simulink model "s8_12"  (Simulink 6.6)
settings: Solver=ode23  SolverMode=SingleTasking  StartTime=0.0  StopTime=t_d  MaxStep=Tc  RelTol=1e-8  AbsTol=1e-8
values from neighbouring files (symbols this model uses):
  F_v = K_r*diag([0.01 0.01])*K_r    [i8_12.m]
  g = 9.81    [i8_12.m]
  K_d = 16*diag([1 1])    [i8_12.m]
  K_p = 100*diag([1 1])    [i8_12.m]
  pi_m = pi_l    [i8_12.m]
  Tc = 0.001    [i8_12.m]
  Ts = Tc    (= 0.001)    [i8_12.m]
undefined symbols (not defined in the file or in its folder): a, iner, iner_l, pi_l, q_i
settings Model: Creator=luigivillani  LastModifiedBy=luigivillani  ExtModeAutoUpdateStatusClock=off
settings SolverCC: InitialStep=0.1*Tc
settings DataIOCC: LimitDataPoints=off  SaveOutput=off  SaveTime=off
settings OptimizationCC: BlockReduction=off  BooleanDataType=off
settings DebuggingCC: SignalResolutionControl=TryResolveAllWithWarning  SolverPrmCheckMsg=none  MultiTaskDSMMsg=warning  MultiTaskCondExecSysMsg=none  StrictBusMsg=None
settings HardwareCC: TargetUnknown=on
settings RTWCC: IncludeERTFirstTime=on

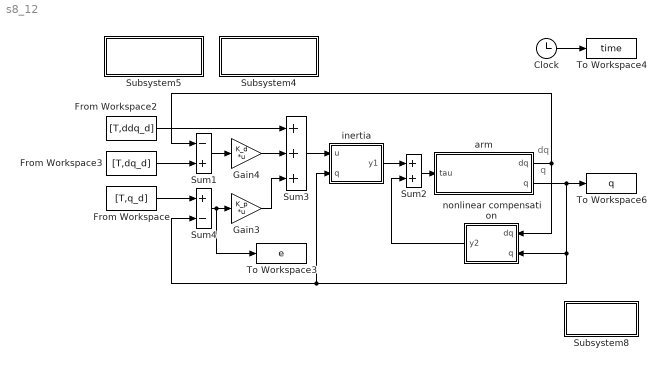
== system s8_12 ==
  note: dq
  note: q
  Clock : Clock
      settings: Decimation=10
  From Workspace : FromWorkspace  VariableName=[T,q_d]  SampleTime=Tc
  From Workspace2 : FromWorkspace  VariableName=[T,ddq_d]  SampleTime=Tc
  From Workspace3 : FromWorkspace  VariableName=[T,dq_d]  SampleTime=Tc
  Gain3 : Gain  Gain=K_p  Multiplication=Matrix(K*u)  SampleTime=Tc
      mask Display: disp('K_p')
  Gain4 : Gain  Gain=K_d  Multiplication=Matrix(K*u)  SampleTime=Tc
      mask Display: disp('K_d')
  Subsystem4 : Subsystem
      settings: OpenFcn=clear all;c=1;i8_12;pi_l=pi_m;
      mask Display: disp('compensated\nload mass')
  Subsystem5 : Subsystem
      settings: OpenFcn=clear all;c=0;i8_12;
      mask Display: disp('noncompensated\nload mass')
  Subsystem8 : Subsystem  Orientation=left
      settings: OpenFcn=p8_12;
      mask Display: disp('plot')
  Sum1 : Sum  Inputs=-+  SampleTime=Tc  SaturateOnIntegerOverflow=on  InputSameDT=on
  Sum2 : Sum  SaturateOnIntegerOverflow=on  InputSameDT=on
  Sum3 : Sum  Inputs=+++  SaturateOnIntegerOverflow=on  InputSameDT=on
  Sum4 : Sum  Inputs=+-  SampleTime=Tc  SaturateOnIntegerOverflow=on  InputSameDT=on
  To Workspace3 : ToWorkspace  VariableName=e  SampleTime=Ts  SaveFormat=Array
      settings: MaxDataPoints=5001
  To Workspace4 : ToWorkspace  VariableName=time  SampleTime=Ts  SaveFormat=Array
      settings: MaxDataPoints=5001
  To Workspace6 : ToWorkspace  VariableName=q  SampleTime=Ts  SaveFormat=Array
      settings: MaxDataPoints=5001
  arm : Subsystem
      mask Display: disp('inv(B(q))(tau-tau'')')
  inertia : Subsystem
      mask Display: disp('B(q)u')
  nonlinear compensation : Subsystem  Orientation=left
      mask Display: disp('n(q,dq)')
  wires:
  Clock/1 -> To Workspace4/1
  Sum2/1 -> arm/1(tau)
  Sum3/1 -> inertia/1(u)
  Gain4/1 -> Sum3/2
  Sum1/1 -> Gain4/1
  From Workspace2/1 -> Sum3/1
  nonlinear compensation/1(y2) -> Sum2/2
  inertia/1(y1) -> Sum2/1
  arm/2("q ") -> To Workspace6/1, Sum4/2, inertia/2(q), nonlinear compensation/2(q)
  From Workspace3/1 -> Sum1/2
  From Workspace/1 -> Sum4/1
  Sum4/1 -> To Workspace3/1, Gain3/1
  arm/1(dq) -> Sum1/1, nonlinear compensation/1(dq)
  Gain3/1 -> Sum3/3

== system s8_12/Subsystem4 ==
  note: start

== system s8_12/Subsystem5 ==
  note: start

== system s8_12/Subsystem8 ==
  note: start

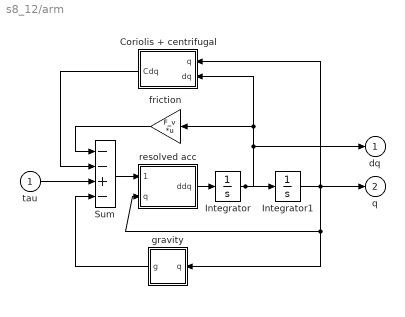
== system s8_12/arm ==
  tau : Inport
  Coriolis + centrifugal : Subsystem  Orientation=left
      mask Display: disp('C(q,dq)dq')
  Integrator : Integrator  InitialCondition=[0 0]  ZeroCross=off
  Integrator1 : Integrator  InitialCondition=q_i  ZeroCross=off
  Sum : Sum  Inputs=--+-  SaturateOnIntegerOverflow=on  InputSameDT=on
  friction : Gain  Orientation=left  Gain=F_v  Multiplication=Matrix(K*u)  SaturateOnIntegerOverflow=on
      mask Display: disp('F_v')
  gravity : Subsystem  Orientation=left
      mask Display: disp('g(q)')
  resolved acc : Subsystem
      mask Display: disp('inv(B(q))')
  dq : Outport  InitialOutput=0
  "q " : Outport  Port=2  InitialOutput=0
  wires:
  Coriolis + centrifugal/1(Cdq) -> Sum/2
  tau/1 -> Sum/3
  Integrator1/1 -> Coriolis + centrifugal/1(q), resolved acc/2(q), gravity/1(q), "q "/1
  resolved acc/1(ddq) -> Integrator/1
  Integrator/1 -> Integrator1/1, dq/1, Coriolis + centrifugal/2(dq), friction/1
  Sum/1 -> resolved acc/1(tau-tau')
  friction/1 -> Sum/1
  gravity/1(g) -> Sum/4

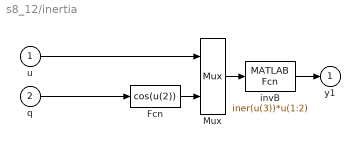
== system s8_12/inertia ==
  u : Inport
  q : Inport  Port=2
  Fcn : Fcn  Expr=cos(u(2))  SampleTime=Tc
  Mux : Mux  Inputs=[2,1]
  "invB " : MATLABFcn  MATLABFcn=iner(u(3))*u(1:2)  OutputDimensions=2  SampleTime=Tc
      mask Display: disp('B(q)')
  y1 : Outport  InitialOutput=0
  wires:
  Fcn/1 -> Mux/2
  "invB "/1 -> y1/1
  Mux/1 -> "invB "/1
  q/1 -> Fcn/1
  u/1 -> Mux/1

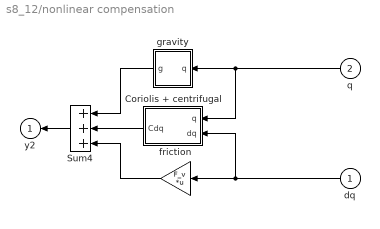
== system s8_12/nonlinear compensation ==
  dq : Inport  Orientation=left
  q : Inport  Orientation=left  Port=2
  Coriolis + centrifugal : Subsystem  Orientation=left
      mask Display: disp('C(q,dq)dq')
  Sum4 : Sum  Orientation=left  Inputs=+++  SaturateOnIntegerOverflow=on  InputSameDT=on
  friction : Gain  Orientation=left  Gain=F_v  Multiplication=Matrix(K*u)  SampleTime=Tc  SaturateOnIntegerOverflow=on
      mask Display: disp('F_v')
  gravity : Subsystem  Orientation=left
      mask Display: disp('g(q)')
  y2 : Outport  Orientation=left  InitialOutput=0
  wires:
  gravity/1(g) -> Sum4/1
  Sum4/1 -> y2/1
  friction/1 -> Sum4/3
  q/1 -> gravity/1(q), Coriolis + centrifugal/1(q)
  dq/1 -> Coriolis + centrifugal/2(dq), friction/1
  Coriolis + centrifugal/1(Cdq) -> Sum4/2

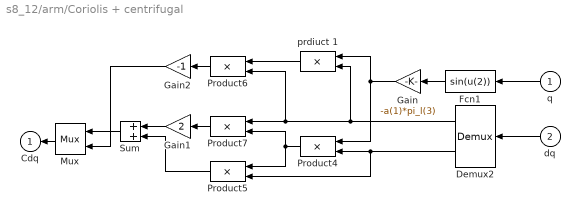
== system s8_12/arm/Coriolis + centrifugal ==
  q : Inport  Orientation=left
  dq : Inport  Orientation=left  Port=2
  Demux2 : Demux  Orientation=left  Outputs=2
  Fcn1 : Fcn  Orientation=left  Expr=sin(u(2))
  Gain : Gain  Orientation=left  Gain=-a(1)*pi_l(3)  SaturateOnIntegerOverflow=on
      mask Display: disp('k_3')
  Gain1 : Gain  Orientation=left  Gain=2  SaturateOnIntegerOverflow=on
  Gain2 : Gain  Orientation=left  Gain=-1  SaturateOnIntegerOverflow=on
  Mux : Mux  Orientation=left  Inputs=2
  Product{4..7} (4 alike) : Product  Orientation=left  SaturateOnIntegerOverflow=on  RndMeth=Zero  InputSameDT=on
  Sum : Sum  Orientation=left  SaturateOnIntegerOverflow=on  InputSameDT=on
  prdiuct 1 : Product  Orientation=left  SaturateOnIntegerOverflow=on  RndMeth=Zero  InputSameDT=on
  Cdq : Outport  Orientation=left  InitialOutput=0
  wires:
  dq/1 -> Demux2/1
  Gain2/1 -> Mux/2
  Product6/1 -> Gain2/1
  Mux/1 -> Cdq/1
  Sum/1 -> Mux/1
  Product5/1 -> Sum/2
  Gain1/1 -> Sum/1
  Product7/1 -> Gain1/1
  Demux2/1 -> prdiuct 1/2, Product6/2, Product7/1
  Demux2/2 -> Product4/2, Product5/2
  prdiuct 1/1 -> Product6/1
  Gain/1 -> prdiuct 1/1, Product4/1
  Fcn1/1 -> Gain/1
  q/1 -> Fcn1/1
  Product4/1 -> Product5/1, Product7/2

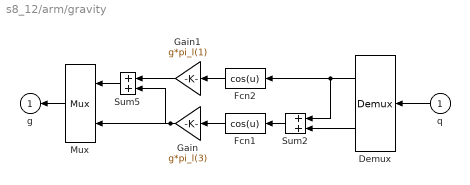
== system s8_12/arm/gravity ==
  q : Inport  Orientation=left
  Demux : Demux  Orientation=left  Outputs=2
  Fcn1 : Fcn  Orientation=left  Expr=cos(u)
  Fcn2 : Fcn  Orientation=left  Expr=cos(u)
  Gain : Gain  Orientation=left  Gain=g*pi_l(3)  SaturateOnIntegerOverflow=on
      mask Display: disp('k_2')
  Gain1 : Gain  Orientation=left  Gain=g*pi_l(1)  SaturateOnIntegerOverflow=on
      mask Display: disp('k_1')
  Mux : Mux  Orientation=left  Inputs=2
  Sum2 : Sum  Orientation=left  SaturateOnIntegerOverflow=on  InputSameDT=on
  Sum5 : Sum  Orientation=left  SaturateOnIntegerOverflow=on  InputSameDT=on
  g : Outport  Orientation=left  InitialOutput=0
  wires:
  q/1 -> Demux/1
  Demux/2 -> Sum2/2
  Sum2/1 -> Fcn1/1
  Fcn1/1 -> Gain/1
  Fcn2/1 -> Gain1/1
  Demux/1 -> Fcn2/1, Sum2/1
  Gain1/1 -> Sum5/1
  Sum5/1 -> Mux/1
  Gain/1 -> Sum5/2, Mux/2
  Mux/1 -> g/1

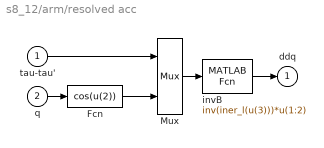
== system s8_12/arm/resolved acc ==
  tau-tau' : Inport
  q : Inport  Port=2
  Fcn : Fcn  Expr=cos(u(2))
  Mux : Mux  Inputs=[2,1]
  "invB " : MATLABFcn  MATLABFcn=inv(iner_l(u(3)))*u(1:2)  OutputDimensions=2
      mask Display: disp('inv(B(q))')
  ddq : Outport  InitialOutput=0
  wires:
  Fcn/1 -> Mux/2
  q/1 -> Fcn/1
  "invB "/1 -> ddq/1
  tau-tau'/1 -> Mux/1
  Mux/1 -> "invB "/1

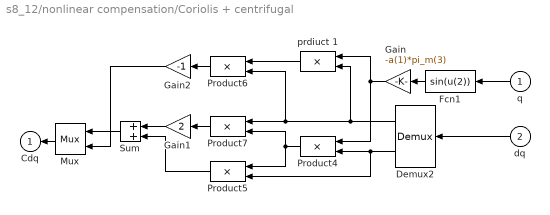
== system s8_12/nonlinear compensation/Coriolis + centrifugal ==
  q : Inport  Orientation=left
  dq : Inport  Orientation=left  Port=2
  Demux2 : Demux  Orientation=left  Outputs=2
  Fcn1 : Fcn  Orientation=left  Expr=sin(u(2))  SampleTime=Tc
  Gain : Gain  Orientation=left  Gain=-a(1)*pi_m(3)  SaturateOnIntegerOverflow=on
      mask Display: disp('k_3')
  Gain1 : Gain  Orientation=left  Gain=2  SaturateOnIntegerOverflow=on
  Gain2 : Gain  Orientation=left  Gain=-1  SaturateOnIntegerOverflow=on
  Mux : Mux  Orientation=left  Inputs=2
  Product{4..7} (4 alike) : Product  Orientation=left  SampleTime=Tc  SaturateOnIntegerOverflow=on  RndMeth=Zero  InputSameDT=on
  Sum : Sum  Orientation=left  SaturateOnIntegerOverflow=on  InputSameDT=on
  prdiuct 1 : Product  Orientation=left  SampleTime=Tc  SaturateOnIntegerOverflow=on  RndMeth=Zero  InputSameDT=on
  Cdq : Outport  Orientation=left  InitialOutput=0
  wires:
  Product4/1 -> Product5/1, Product7/2
  Demux2/1 -> prdiuct 1/2, Product6/2, Product7/1
  Fcn1/1 -> Gain/1
  Gain/1 -> prdiuct 1/1, Product4/1
  prdiuct 1/1 -> Product6/1
  Product7/1 -> Gain1/1
  Gain1/1 -> Sum/1
  Product5/1 -> Sum/2
  Sum/1 -> Mux/1
  Mux/1 -> Cdq/1
  Product6/1 -> Gain2/1
  Gain2/1 -> Mux/2
  q/1 -> Fcn1/1
  dq/1 -> Demux2/1
  Demux2/2 -> Product4/2, Product5/2

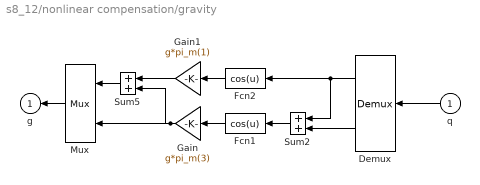
== system s8_12/nonlinear compensation/gravity ==
  q : Inport  Orientation=left
  Demux : Demux  Orientation=left  Outputs=2
  Fcn1 : Fcn  Orientation=left  Expr=cos(u)  SampleTime=Tc
  Fcn2 : Fcn  Orientation=left  Expr=cos(u)  SampleTime=Tc
  Gain : Gain  Orientation=left  Gain=g*pi_m(3)  SaturateOnIntegerOverflow=on
      mask Display: disp('k_2')
  Gain1 : Gain  Orientation=left  Gain=g*pi_m(1)  SaturateOnIntegerOverflow=on
      mask Display: disp('k_1')
  Mux : Mux  Orientation=left  Inputs=2
  Sum2 : Sum  Orientation=left  SampleTime=Tc  SaturateOnIntegerOverflow=on  InputSameDT=on
  Sum5 : Sum  Orientation=left  SaturateOnIntegerOverflow=on  InputSameDT=on
  g : Outport  Orientation=left  InitialOutput=0
  wires:
  q/1 -> Demux/1
  Demux/2 -> Sum2/2
  Sum2/1 -> Fcn1/1
  Fcn1/1 -> Gain/1
  Fcn2/1 -> Gain1/1
  Demux/1 -> Fcn2/1, Sum2/1
  Gain1/1 -> Sum5/1
  Sum5/1 -> Mux/1
  Gain/1 -> Mux/2, Sum5/2
  Mux/1 -> g/1
